simulink model "sim_velo_control_PI_zeta_omega"  (R2021b)
settings: Solver=ode1  StartTime=0.0  StopTime=1  FixedStep=0.01  RelTol=1e-3
values from neighbouring files (symbols this model uses):
  a = 27.65    [motor_parameter_and_pole_calculate.m]
  b = 17.35    [motor_parameter_and_pole_calculate.m]
  ki = wn^2/b    (= 81.9148722626)    [motor_parameter_and_pole_calculate.m]
  kp = (2*zeta*wn-a)/b    (= 2.75205900208)    [motor_parameter_and_pole_calculate.m]
  wnf = 2*pi*10    (= 62.8318530718)    [motor_parameter_and_pole_calculate.m]
  zetaf = 1    [motor_parameter_and_pole_calculate.m]
libraries: slpidlib x3
settings Model: Creator=ONLY-GOD  LastModifiedBy=ASUS
settings SolverCC: AlgebraicLoopSolver=TrustRegion
settings DebuggingCC: SFMachineParentedDataDiag=warning

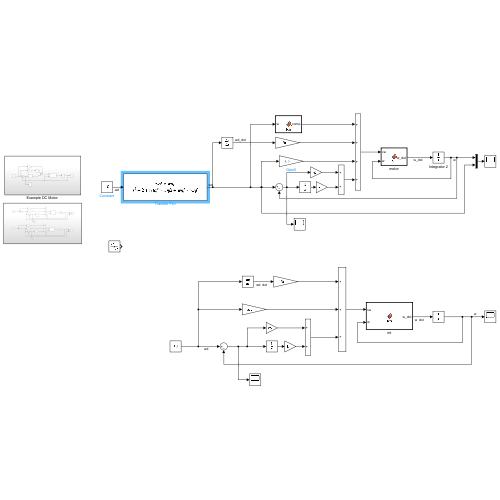
[thumbnail: Simulink's stored preview of the top-level diagram]
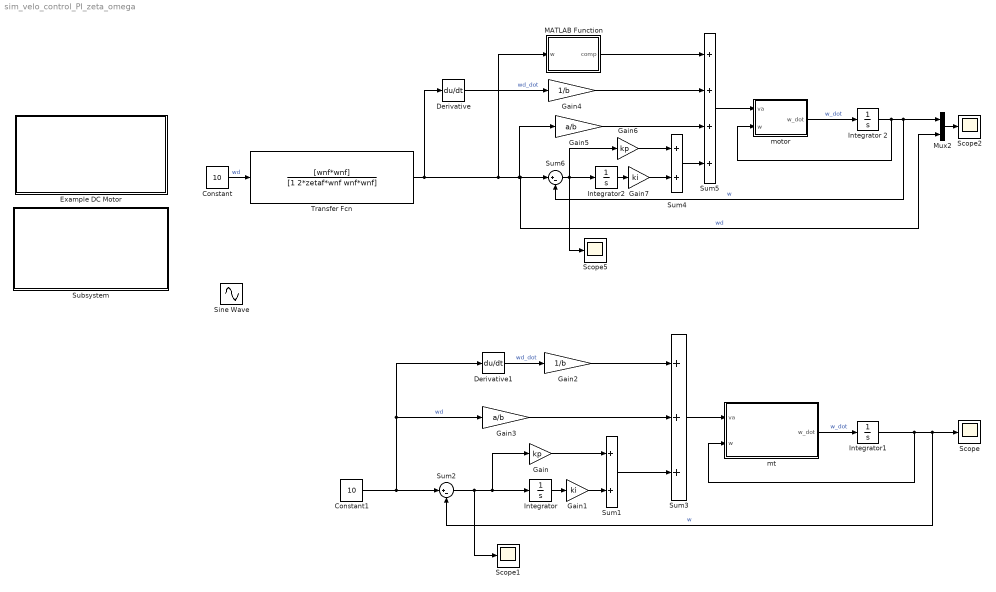
== system sim_velo_control_PI_zeta_omega ==
  Constant : Constant  Value=10
  Constant1 : Constant  Value=10
  Derivative : Derivative
  Derivative1 : Derivative
  "Example DC Motor " : Subsystem
  Gain : Gain  Gain=kp
  Gain1 : Gain  Gain=ki
  Gain2 : Gain  Gain=1/b
  Gain3 : Gain  Gain=a/b
  Gain4 : Gain  Gain=1/b
  Gain5 : Gain  Gain=a/b
  Gain6 : Gain  Gain=kp
  Gain7 : Gain  Gain=ki
  Integrator : Integrator
  Integrator 2 : Integrator
  Integrator1 : Integrator
  Integrator2 : Integrator
  MATLAB Function : MATLAB Function  TreatAsAtomicUnit=on
  Mux2 : Mux  Inputs=2
  Scope{,1..2,5} (4 alike) : Scope
  Sine Wave : Sin  Amplitude=10  Frequency=2*pi*0.1  SampleTime=0
  Subsystem : Subsystem
  Sum1 : Sum
  Sum2 : Sum  Inputs=|+-
  Sum3 : Sum  Inputs=+++
  Sum4 : Sum
  Sum5 : Sum  Inputs=++++
  Sum6 : Sum  Inputs=|+-
  Transfer Fcn : TransferFcn  Numerator=[wnf*wnf]  Denominator=[1 2*zetaf*wnf wnf*wnf]
  motor : MATLAB Function  TreatAsAtomicUnit=on
  mt : MATLAB Function  TreatAsAtomicUnit=on
  wires:
  Gain5/1 -> Sum5/3
  Mux2/1 -> Scope2/1
  Sum5/1 -> motor/1(va)
  Integrator 2/1 -> motor/2(w), Sum6/2, Mux2/1  "w"
  motor/1(w_dot) -> Integrator 2/1  "w_dot"
  Gain4/1 -> Sum5/2
  Transfer Fcn/1 -> Derivative/1, MATLAB Function/1(w), Gain5/1, Mux2/2, Sum6/1  "wd"
  MATLAB Function/1(comp) -> Sum5/1
  Derivative/1 -> Gain4/1  "wd_dot"
  Integrator/1 -> Gain1/1
  Gain/1 -> Sum1/1
  Gain1/1 -> Sum1/2
  Sum2/1 -> Scope1/1, Integrator/1, Gain/1
  Sum1/1 -> Sum3/3
  Gain2/1 -> Sum3/1
  Gain3/1 -> Sum3/2
  Derivative1/1 -> Gain2/1  "wd_dot"
  Sum3/1 -> mt/1(va)
  mt/1(w_dot) -> Integrator1/1  "w_dot"
  Integrator1/1 -> Sum2/2, Scope/1, mt/2(w)  "w"
  Constant1/1 -> Derivative1/1, Gain3/1, Sum2/1  "wd"
  Gain6/1 -> Sum4/1
  Gain7/1 -> Sum4/2
  Integrator2/1 -> Gain7/1
  Sum4/1 -> Sum5/4
  Sum6/1 -> Gain6/1, Integrator2/1, Scope5/1
  Constant/1 -> Transfer Fcn/1  "wd"

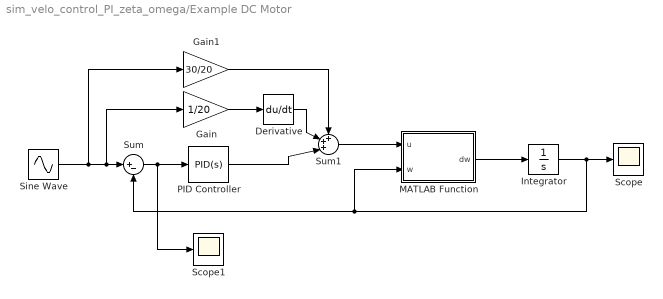
== system sim_velo_control_PI_zeta_omega/Example DC Motor  ==
  Derivative : Derivative
  Gain : Gain  Gain=1/20
  Gain1 : Gain  Gain=30/20
  Integrator : Integrator
  MATLAB Function : MATLAB Function  TreatAsAtomicUnit=on
  PID Controller : slpidlib/PID Controller  Controller=PID  Form=Parallel  TimeDomain=Continuous-time  UseExternalTs=off  SampleTime=-1  IntegratorMethod=Forward Euler  FilterMethod=Forward Euler  ControllerParametersSource=internal  P=1.5  I=71  D=0  UseFilter=on  N=100  TunerSelectOption=Transfer Function Based (PID Tuner App)  InitialConditionSource=internal  InitialConditionForIntegrator=0  InitialConditionForFilter=0  DifferentiatorICPrevScaledInput=0  ExternalReset=none  TrackingMode=off  Kt=1  LimitOutput=off  SatLimitsSource=internal  UpperSaturationLimit=inf  LowerSaturationLimit=-inf  LinearizeAsGain=on  AntiWindupMode=none  Kb=1  POutMin=[]  POutMax=[]  IOutMin=[]  IOutMax=[]  DOutMin=[]  DOutMax=[]  NOutMin=[]  NOutMax=[]  SumOutMin=[]  SumOutMax=[]  SaturationOutMin=[]  SaturationOutMax=[]  PParamMin=[]  PParamMax=[]  IParamMin=[]  IParamMax=[]  DParamMin=[]  DParamMax=[]  NParamMin=[]  NParamMax=[]  KbParamMin=[]  KbParamMax=[]  KtParamMin=[]  KtParamMax=[]  KbOutMin=[]  KbOutMax=[]  KtOutMin=[]  KtOutMax=[]  IntegratorOutMin=[]  IntegratorOutMax=[]  FilterOutMin=[]  FilterOutMax=[]  SumI1OutMin=[]  SumI1OutMax=[]  SumI2OutMin=[]  SumI2OutMax=[]  SumI3OutMin=[]  SumI3OutMax=[]  SumI4OutMin=[]  SumI4OutMax=[]  SumDOutMin=[]  SumDOutMax=[]  DifferentiatorOutMin=[]  DifferentiatorOutMax=[]  FilterDiffOutCoefMin=[]  FilterDiffOutCoefMax=[]  ReciprocalOutMin=[]  ReciprocalOutMax=[]  SumDenOutMin=[]  SumDenOutMax=[]  SumNumOutMin=[]  SumNumOutMax=[]  DivideOutMin=[]  DivideOutMax=[]  UdiffTsProdOutMin=[]  UdiffTsProdOutMax=[]  NTsProdOutMin=[]  NTsProdOutMax=[]  UintegralTsProdOutMin=[]  UintegralTsProdOutMax=[]  UngainTsProdOutMin=[]  UngainTsProdOutMax=[]  IntegratorContinuousStateAttributes=''  IntegratorStateMustResolveToSignalObject=off  IntegratorRTWStateStorageClass=Auto  FilterContinuousStateAttributes=''  FilterStateMustResolveToSignalObject=off  FilterRTWStateStorageClass=Auto  ParallelPVariant=InternalParameters  IdealPVariant=Disabled  IVariant=InternalParameters  DVariant=InternalParameters  IntegratorVariant=Continuous  SatVariant=Disabled  AWVariant=Passthrough  PCopyVariant=Disabled  TRVariant=Disabled  FdbkBlocksVariant=Forward  IdealPFdbkVariant=Disabled  SatFdbkVariant=Disabled  DerivativeFilterVariant=ContFilter  NVariant=InternalParameters  NCopyVariant=Disabled  FilterICVariant=InternalICsFilter  IntegratorICVariant=InternalICs  ExternalResetVariant=Disabled  TRSumVariant=Passthrough  SumFdbkVariant=Disabled  SumVariant=Sum_PID  TsampFilterVariant=InternalTs  TsampNgainVariant=Passthrough  TsampIntegralVariant=Passthrough  ExternalSaturationOutDataTypeStr=Inherit: Same as second input
  Scope : Scope
  Scope1 : Scope
  Sine Wave : Sin  Amplitude=10  SampleTime=0
  Sum : Sum  Inputs=|+-
  Sum1 : Sum  Inputs=+++|
  wires:
  Integrator/1 -> Scope/1, MATLAB Function/2(w), Sum/2
  MATLAB Function/1(dw) -> Integrator/1
  Gain/1 -> Derivative/1
  Sum1/1 -> MATLAB Function/1(u)
  Sum/1 -> Scope1/1, PID Controller/1
  Sine Wave/1 -> Gain1/1, Gain/1, Sum/1
  Derivative/1 -> Sum1/2
  PID Controller/1 -> Sum1/3
  Gain1/1 -> Sum1/1

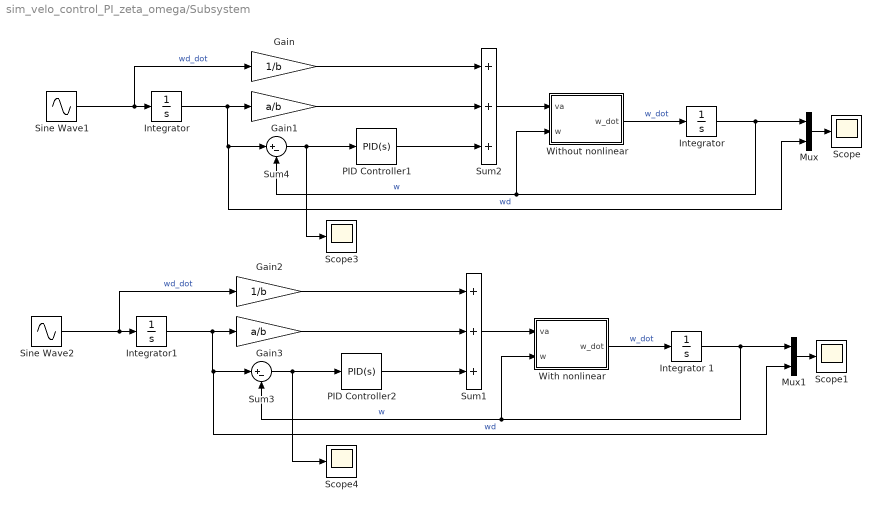
== system sim_velo_control_PI_zeta_omega/Subsystem ==
  Gain : Gain  Gain=1/b
  Gain1 : Gain  Gain=a/b
  Gain2 : Gain  Gain=1/b
  Gain3 : Gain  Gain=a/b
  Integrator : Integrator
  "Integrator " : Integrator
  Integrator 1 : Integrator
  Integrator1 : Integrator
  Mux : Mux  Inputs=2
  Mux1 : Mux  Inputs=2
  PID Controller1 : slpidlib/PID Controller  Controller=PID  Form=Parallel  TimeDomain=Continuous-time  UseExternalTs=off  SampleTime=-1  IntegratorMethod=Forward Euler  FilterMethod=Forward Euler  ControllerParametersSource=internal  P=kp  I=ki  D=0  UseFilter=on  N=100  TunerSelectOption=Transfer Function Based (PID Tuner App)  InitialConditionSource=internal  InitialConditionForIntegrator=0  InitialConditionForFilter=0  DifferentiatorICPrevScaledInput=0  ExternalReset=none  TrackingMode=off  Kt=1  LimitOutput=off  SatLimitsSource=internal  UpperSaturationLimit=inf  LowerSaturationLimit=-inf  LinearizeAsGain=on  AntiWindupMode=none  Kb=1  POutMin=[]  POutMax=[]  IOutMin=[]  IOutMax=[]  DOutMin=[]  DOutMax=[]  NOutMin=[]  NOutMax=[]  SumOutMin=[]  SumOutMax=[]  SaturationOutMin=[]  SaturationOutMax=[]  PParamMin=[]  PParamMax=[]  IParamMin=[]  IParamMax=[]  DParamMin=[]  DParamMax=[]  NParamMin=[]  NParamMax=[]  KbParamMin=[]  KbParamMax=[]  KtParamMin=[]  KtParamMax=[]  KbOutMin=[]  KbOutMax=[]  KtOutMin=[]  KtOutMax=[]  IntegratorOutMin=[]  IntegratorOutMax=[]  FilterOutMin=[]  FilterOutMax=[]  SumI1OutMin=[]  SumI1OutMax=[]  SumI2OutMin=[]  SumI2OutMax=[]  SumI3OutMin=[]  SumI3OutMax=[]  SumI4OutMin=[]  SumI4OutMax=[]  SumDOutMin=[]  SumDOutMax=[]  DifferentiatorOutMin=[]  DifferentiatorOutMax=[]  FilterDiffOutCoefMin=[]  FilterDiffOutCoefMax=[]  ReciprocalOutMin=[]  ReciprocalOutMax=[]  SumDenOutMin=[]  SumDenOutMax=[]  SumNumOutMin=[]  SumNumOutMax=[]  DivideOutMin=[]  DivideOutMax=[]  UdiffTsProdOutMin=[]  UdiffTsProdOutMax=[]  NTsProdOutMin=[]  NTsProdOutMax=[]  UintegralTsProdOutMin=[]  UintegralTsProdOutMax=[]  UngainTsProdOutMin=[]  UngainTsProdOutMax=[]  IntegratorContinuousStateAttributes=''  IntegratorStateMustResolveToSignalObject=off  IntegratorRTWStateStorageClass=Auto  FilterContinuousStateAttributes=''  FilterStateMustResolveToSignalObject=off  FilterRTWStateStorageClass=Auto  ParallelPVariant=InternalParameters  IdealPVariant=Disabled  IVariant=InternalParameters  DVariant=InternalParameters  IntegratorVariant=Continuous  SatVariant=Disabled  AWVariant=Passthrough  PCopyVariant=Disabled  TRVariant=Disabled  FdbkBlocksVariant=Forward  IdealPFdbkVariant=Disabled  SatFdbkVariant=Disabled  DerivativeFilterVariant=ContFilter  NVariant=InternalParameters  NCopyVariant=Disabled  FilterICVariant=InternalICsFilter  IntegratorICVariant=InternalICs  ExternalResetVariant=Disabled  TRSumVariant=Passthrough  SumFdbkVariant=Disabled  SumVariant=Sum_PID  TsampFilterVariant=InternalTs  TsampNgainVariant=Passthrough  TsampIntegralVariant=Passthrough  ExternalSaturationOutDataTypeStr=Inherit: Same as second input
  PID Controller2 : slpidlib/PID Controller  Controller=PID  Form=Parallel  TimeDomain=Continuous-time  UseExternalTs=off  SampleTime=-1  IntegratorMethod=Forward Euler  FilterMethod=Forward Euler  ControllerParametersSource=internal  P=kp  I=ki  D=0  UseFilter=on  N=100  TunerSelectOption=Transfer Function Based (PID Tuner App)  InitialConditionSource=internal  InitialConditionForIntegrator=0  InitialConditionForFilter=0  DifferentiatorICPrevScaledInput=0  ExternalReset=none  TrackingMode=off  Kt=1  LimitOutput=off  SatLimitsSource=internal  UpperSaturationLimit=inf  LowerSaturationLimit=-inf  LinearizeAsGain=on  AntiWindupMode=none  Kb=1  POutMin=[]  POutMax=[]  IOutMin=[]  IOutMax=[]  DOutMin=[]  DOutMax=[]  NOutMin=[]  NOutMax=[]  SumOutMin=[]  SumOutMax=[]  SaturationOutMin=[]  SaturationOutMax=[]  PParamMin=[]  PParamMax=[]  IParamMin=[]  IParamMax=[]  DParamMin=[]  DParamMax=[]  NParamMin=[]  NParamMax=[]  KbParamMin=[]  KbParamMax=[]  KtParamMin=[]  KtParamMax=[]  KbOutMin=[]  KbOutMax=[]  KtOutMin=[]  KtOutMax=[]  IntegratorOutMin=[]  IntegratorOutMax=[]  FilterOutMin=[]  FilterOutMax=[]  SumI1OutMin=[]  SumI1OutMax=[]  SumI2OutMin=[]  SumI2OutMax=[]  SumI3OutMin=[]  SumI3OutMax=[]  SumI4OutMin=[]  SumI4OutMax=[]  SumDOutMin=[]  SumDOutMax=[]  DifferentiatorOutMin=[]  DifferentiatorOutMax=[]  FilterDiffOutCoefMin=[]  FilterDiffOutCoefMax=[]  ReciprocalOutMin=[]  ReciprocalOutMax=[]  SumDenOutMin=[]  SumDenOutMax=[]  SumNumOutMin=[]  SumNumOutMax=[]  DivideOutMin=[]  DivideOutMax=[]  UdiffTsProdOutMin=[]  UdiffTsProdOutMax=[]  NTsProdOutMin=[]  NTsProdOutMax=[]  UintegralTsProdOutMin=[]  UintegralTsProdOutMax=[]  UngainTsProdOutMin=[]  UngainTsProdOutMax=[]  IntegratorContinuousStateAttributes=''  IntegratorStateMustResolveToSignalObject=off  IntegratorRTWStateStorageClass=Auto  FilterContinuousStateAttributes=''  FilterStateMustResolveToSignalObject=off  FilterRTWStateStorageClass=Auto  ParallelPVariant=InternalParameters  IdealPVariant=Disabled  IVariant=InternalParameters  DVariant=InternalParameters  IntegratorVariant=Continuous  SatVariant=Disabled  AWVariant=Passthrough  PCopyVariant=Disabled  TRVariant=Disabled  FdbkBlocksVariant=Forward  IdealPFdbkVariant=Disabled  SatFdbkVariant=Disabled  DerivativeFilterVariant=ContFilter  NVariant=InternalParameters  NCopyVariant=Disabled  FilterICVariant=InternalICsFilter  IntegratorICVariant=InternalICs  ExternalResetVariant=Disabled  TRSumVariant=Passthrough  SumFdbkVariant=Disabled  SumVariant=Sum_PID  TsampFilterVariant=InternalTs  TsampNgainVariant=Passthrough  TsampIntegralVariant=Passthrough  ExternalSaturationOutDataTypeStr=Inherit: Same as second input
  Scope{,1,3..4} (4 alike) : Scope
  Sine Wave1 : Sin  Amplitude=10  Frequency=2*pi*0.1  SampleTime=0
  Sine Wave2 : Sin  Amplitude=10  Frequency=2*pi*0.1  SampleTime=0
  Sum1 : Sum  Inputs=+++
  Sum2 : Sum  Inputs=+++
  Sum3 : Sum  Inputs=|+-
  Sum4 : Sum  Inputs=|+-
  With nonlinear : MATLAB Function  TreatAsAtomicUnit=on
  "Without nonlinear " : MATLAB Function  TreatAsAtomicUnit=on
  wires:
  Sine Wave2/1 -> Gain2/1, Integrator1/1  "wd_dot"
  PID Controller1/1 -> Sum2/3
  "Integrator "/1 -> Mux/1, Sum4/2, "Without nonlinear "/2(w)  "w"
  Gain1/1 -> Sum2/2
  Integrator/1 -> Mux/2, Sum4/1, Gain1/1  "wd"
  Sum2/1 -> "Without nonlinear "/1(va)
  "Without nonlinear "/1(w_dot) -> "Integrator "/1  "w_dot"
  Sum3/1 -> Scope4/1, PID Controller2/1
  Integrator 1/1 -> With nonlinear/2(w), Sum3/2, Mux1/1  "w"
  Mux1/1 -> Scope1/1
  Integrator1/1 -> Gain3/1, Sum3/1, Mux1/2  "wd"
  Sine Wave1/1 -> Integrator/1, Gain/1  "wd_dot"
  Gain2/1 -> Sum1/1
  Gain3/1 -> Sum1/2
  PID Controller2/1 -> Sum1/3
  Gain/1 -> Sum2/1
  With nonlinear/1(w_dot) -> Integrator 1/1  "w_dot"
  Sum4/1 -> Scope3/1, PID Controller1/1
  Sum1/1 -> With nonlinear/1(va)
  Mux/1 -> Scope/1

== matlab function sim_velo_control_PI_zeta_omega/Example DC Motor /MATLAB Function ==
  settings: updateMethod=DISCRETE
  data: u input; dw output; w input
function dw = dcmotor(u,w)

a = 30; b = 20; c = 5.63;
dw = -a*w + b*u;

== matlab function sim_velo_control_PI_zeta_omega/Subsystem/Without nonlinear  ==
  data: va input; w_dot output; w input
function w_dot = fcn(va,w)
%#codegen
a = 27.65;
b = 17.35;
c = 5.635;
w_dot = -a*w + b*va;% -c*sign(w);

== matlab function sim_velo_control_PI_zeta_omega/motor ==
  data: va input; w_dot output; w input
function w_dot = fcn(va,w)
%#codegen
a = 27.65;
b = 17.35;
c = 5.635;
w_dot = -a*w + b*va -c*sign(w);

== matlab function sim_velo_control_PI_zeta_omega/MATLAB Function ==
  data: w input; comp output
function comp = fcn(w)
a = 27.65;
b = 17.35;
c = 5.635;

comp = -(c/b)*sign(w);

== matlab function sim_velo_control_PI_zeta_omega/mt ==
  data: va input; w_dot output; w input
function w_dot = fcn(va,w)
%#codegen
a = 27.65;
b = 17.35;
c = 5.635;
w_dot = -a*w + b*va -c*sign(w);

== matlab function sim_velo_control_PI_zeta_omega/Subsystem/With nonlinear ==
  data: va input; w_dot output; w input
function w_dot = fcn(va,w)
%#codegen
a = 27.65;
b = 17.35;
c = 5.635;
w_dot = -a*w + b*va -c*sign(w);
